simulink model "GasTurbinePropulsion"  (Simulink 8.3)
settings: Solver=ode45  StartTime=0.0  StopTime=10.0  RelTol=1e-3
undefined symbols (not defined in the file): sigbuilder_block
libraries: simulink_need_slupdate x1
(part 2 of 2)

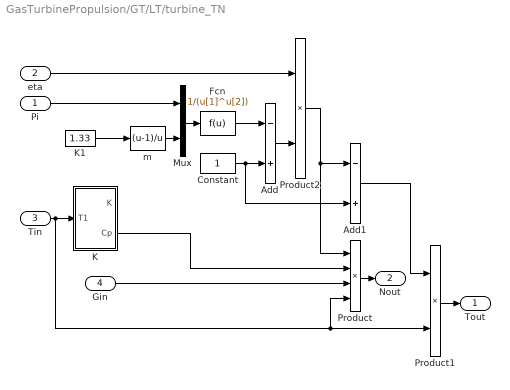
== system GasTurbinePropulsion/GT/LT/turbine_TN ==
  Pi : Inport
  eta : Inport  Port=2
  Tin : Inport  Port=3
  Gin : Inport  Port=4
  Add : Sum  Inputs=-+
  Add1 : Sum  Inputs=-+
  Constant : Constant
  Fcn : Fcn  Expr=1/(u[1]^u[2])
  K : Subsystem
  K1 : Constant  Value=1.33
  Mux : Mux  Inputs=2
  Product : Product  Inputs=4  RndMeth=Zero
  Product1 : Product  RndMeth=Zero
  Product2 : Product  RndMeth=Zero
  m : Fcn  Expr=(u-1)/u
  Tout : Outport
  Nout : Outport  Port=2
  wires:
  Tin/1 -> K/1(T1), Product1/2, Product/4
  Pi/1 -> Mux/1
  m/1 -> Mux/2
  Mux/1 -> Fcn/1
  Fcn/1 -> Add/1
  Add/1 -> Product2/2
  eta/1 -> Product2/1
  Product2/1 -> Add1/1, Product/1
  Constant/1 -> Add/2, Add1/2
  Product1/1 -> Tout/1
  Product/1 -> Nout/1
  Add1/1 -> Product1/1
  K/2(Cp) -> Product/2
  Gin/1 -> Product/3
  K1/1 -> m/1

== system GasTurbinePropulsion/GT/PT/turbine_TN ==
  Pi : Inport
  eta : Inport  Port=2
  Gin : Inport  Port=3
  Tin : Inport  Port=4
  Add : Sum  Inputs=-+
  Add1 : Sum  Inputs=-+
  Constant : Constant
  Fcn : Fcn  Expr=1/(u[1]^u[2])
  K1 : Subsystem
  Mux : Mux  Inputs=2
  Product : Product  Inputs=4  RndMeth=Zero
  Product1 : Product  RndMeth=Zero
  Product2 : Product  RndMeth=Zero
  m : Fcn  Expr=(u-1)/u
  Tout : Outport
  Nout : Outport  Port=2
  wires:
  Pi/1 -> Mux/1
  m/1 -> Mux/2
  Mux/1 -> Fcn/1
  Fcn/1 -> Add/1
  Add/1 -> Product2/2
  eta/1 -> Product2/1
  Product2/1 -> Add1/1, Product/1
  Constant/1 -> Add/2, Add1/2
  Product1/1 -> Tout/1
  Product/1 -> Nout/1
  Add1/1 -> Product1/1
  Gin/1 -> Product/3
  Tin/1 -> K1/1(T1), Product1/2, Product/4
  K1/2(Cp) -> Product/2
  K1/1(K) -> m/1

== system GasTurbinePropulsion/GT/HC/compresser_TN/K ==
  note: Cv
  note: Cp
  T1 : Inport
  Add : Sum
  Add1 : Sum
  Add2 : Sum  Inputs=+-
  Constant : Constant  Value=0.9956
  Constant1 : Constant  Value=0.7088
  Divide1 : Product  Inputs=*/
  Gain2 : Gain  Gain=0.000093
  Gain3 : Gain  Gain=0.000093
  Scope3 : Scope
      settings: YMin=2829.54  YMax=3127.38  SaveName=ScopeData23
  Tk : Constant  Value=273.15
  K : Outport
  Cp : Outport  Port=2
  wires:
  Divide1/1 -> K/1, Scope3/1
  Add1/1 -> Divide1/2
  Constant1/1 -> Add1/2
  Gain3/1 -> Add1/1
  Add/1 -> Divide1/1, Cp/1
  Constant/1 -> Add/2
  Gain2/1 -> Add/1
  T1/1 -> Add2/1
  Tk/1 -> Add2/2
  Add2/1 -> Gain2/1, Gain3/1

== system GasTurbinePropulsion/GT/HT/turbine_TN/K ==
  note: Cv
  note: Cp
  T1 : Inport
  Add : Sum
  Add1 : Sum
  Add2 : Sum  Inputs=+-
  Constant : Constant  Value=0.9956
  Constant1 : Constant  Value=0.7088
  Divide1 : Product  Inputs=*/
  Gain2 : Gain  Gain=0.000093
  Gain3 : Gain  Gain=0.000093
  Tk : Constant  Value=273.15
  K : Outport
  Cp : Outport  Port=2
  wires:
  Divide1/1 -> K/1
  Add1/1 -> Divide1/2
  Constant1/1 -> Add1/2
  Gain3/1 -> Add1/1
  Add/1 -> Divide1/1, Cp/1
  Constant/1 -> Add/2
  Gain2/1 -> Add/1
  T1/1 -> Add2/1
  Tk/1 -> Add2/2
  Add2/1 -> Gain2/1, Gain3/1

== system GasTurbinePropulsion/GT/LC/compresser_TN/K ==
  note: Cv
  note: Cp
  T1 : Inport
  Add : Sum
  Add1 : Sum
  Add2 : Sum  Inputs=+-
  Constant : Constant  Value=0.9956
  Constant1 : Constant  Value=0.7088
  Divide1 : Product  Inputs=*/
  Gain2 : Gain  Gain=0.000093
  Gain3 : Gain  Gain=0.000093
  Tk : Constant  Value=273.15
  K : Outport
  Cp : Outport  Port=2
  wires:
  Divide1/1 -> K/1
  Add1/1 -> Divide1/2
  Constant1/1 -> Add1/2
  Gain3/1 -> Add1/1
  Add/1 -> Divide1/1, Cp/1
  Constant/1 -> Add/2
  Gain2/1 -> Add/1
  T1/1 -> Add2/1
  Tk/1 -> Add2/2
  Add2/1 -> Gain2/1, Gain3/1

== system GasTurbinePropulsion/GT/LT/turbine_TN/K ==
  note: Cv
  note: Cp
  T1 : Inport
  Add : Sum
  Add1 : Sum
  Add2 : Sum  Inputs=+-
  Constant : Constant  Value=0.9956
  Constant1 : Constant  Value=0.7088
  Divide1 : Product  Inputs=*/
  Gain2 : Gain  Gain=0.000093
  Gain3 : Gain  Gain=0.000093
  Tk : Constant  Value=273.15
  K : Outport
  Cp : Outport  Port=2
  wires:
  Divide1/1 -> K/1
  Add1/1 -> Divide1/2
  Constant1/1 -> Add1/2
  Gain3/1 -> Add1/1
  Add/1 -> Divide1/1, Cp/1
  Constant/1 -> Add/2
  Gain2/1 -> Add/1
  T1/1 -> Add2/1
  Tk/1 -> Add2/2
  Add2/1 -> Gain2/1, Gain3/1

== system GasTurbinePropulsion/GT/PT/turbine_TN/K1 ==
  note: Cp
  note: Cv
  T1 : Inport
  Add : Sum
  Add1 : Sum
  Add2 : Sum  Inputs=+-
  Constant : Constant  Value=0.9956
  Constant1 : Constant  Value=0.7088
  Divide1 : Product  Inputs=*/
  Gain2 : Gain  Gain=0.000093
  Gain3 : Gain  Gain=0.000093
  Tk : Constant  Value=273.15
  K : Outport
  Cp : Outport  Port=2
  wires:
  Add/1 -> Divide1/1, Cp/1
  Constant/1 -> Add/2
  Gain2/1 -> Add/1
  T1/1 -> Add2/1
  Tk/1 -> Add2/2
  Add2/1 -> Gain2/1, Gain3/1
  Divide1/1 -> K/1
  Add1/1 -> Divide1/2
  Constant1/1 -> Add1/2
  Gain3/1 -> Add1/1

== matlab function propeller/Embedded MATLAB Function1 ==
  data: u input double; y output double; u1 input double
function y = fcn(u,u1)
% This block supports the Embedded MATLAB subset.
% See the help menu for details. 

if u>0 u1>0
    y=0.1
elseif u=0 u1=0
        y=0
else y=0.25

== matlab function propeller/Embedded MATLAB Function ==
  data: u input double; y output double
function y = fcn(u)
% This block supports the Embedded MATLAB subset.
% See the help menu for details. 

if u<=-1
    y=3
elseif u<=0
    y=(-3)*u
elseif u<1
    y=u
else
    y=1
end
